simulink model "DCMotorSpeedControl_ClosedLoop"  (R2015b)
settings: Solver=VariableStepAuto  StartTime=0.0  StopTime=5  RelTol=1e-3
values from neighbouring files (symbols this model uses):
  Kv = (Vdc_nom - (I_nl*R_winding))/Om_nl    (= 0.00375385553259)    [MotorModel_Mabuchi_RS_540.m]    (also in Params.m = 0.0039)
  Vdc = 9.6    [MotorModel_Mabuchi_RS_540.m]    (also in Params.m)
libraries: LocalLib x2, simulink x1
settings Model: Creator=jje  LastModifiedBy=jje

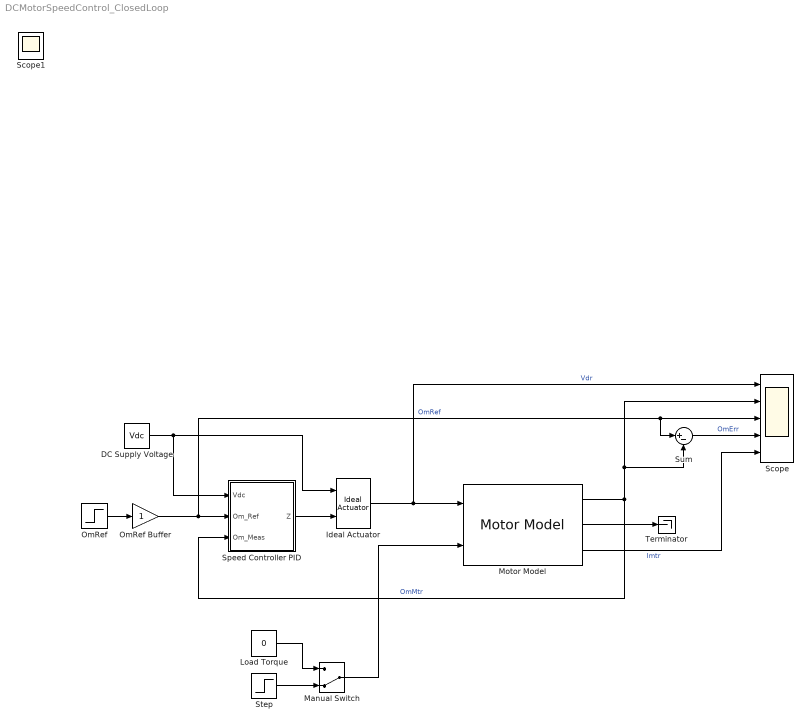
== system DCMotorSpeedControl_ClosedLoop ==
  DC Supply Voltage : Constant  Value=Vdc
  Ideal Actuator : LocalLib/Ideal Actuator
  Load Torque : Constant  Value=0
  Manual Switch : ManualSwitch  CurrentSetting=0
  Motor Model : LocalLib/Motor Model
  OmRef : Step  Time=0.01  After=10000*2*pi/60  SampleTime=0
  OmRef Buffer : Gain
  Scope : Scope  NumInputPorts=5
  Speed Controller PID : Subsystem
  Step : Step  Time=2  After=-0.1  SampleTime=0
  Sum : Sum  Inputs=|+-
  Terminator : Terminator
  Scope1 : Scope
  wires:
  DC Supply Voltage/1 -> Speed Controller PID/1(Vdc), Ideal Actuator/1
  Ideal Actuator/1 -> Motor Model/1, Scope/1  "Vdr"
  Motor Model/1 -> Speed Controller PID/3(Om_Meas), Sum/2, Scope/2  "OmMtr"
  Manual Switch/1 -> Motor Model/2
  OmRef/1 -> OmRef Buffer/1
  OmRef Buffer/1 -> Sum/1, Scope/3, Speed Controller PID/2(Om_Ref)  "OmRef"
  Sum/1 -> Scope/4  "OmErr"
  Motor Model/3 -> Scope/5  "Imtr"
  Motor Model/2 -> Terminator/1
  Speed Controller PID/1(Z) -> Ideal Actuator/2
  Load Torque/1 -> Manual Switch/1
  Step/1 -> Manual Switch/2

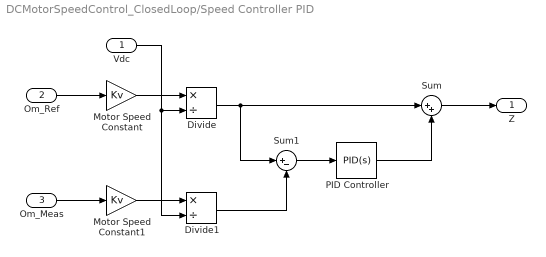
== system DCMotorSpeedControl_ClosedLoop/Speed Controller PID ==
  Vdc : Inport
  Om_Ref : Inport  Port=2
  Om_Meas : Inport  Port=3
  Divide : Product  Inputs=*/
  Divide1 : Product  Inputs=*/
  Motor Speed Constant : Gain  Gain=Kv
  Motor Speed Constant1 : Gain  Gain=Kv
  PID Controller : simulink/Continuous/PID Controller  Controller=PID  TimeDomain=Continuous-time  SampleTime=-1  IntegratorMethod=Forward Euler  FilterMethod=Forward Euler  Form=Ideal  UseFilter=on  ControllerParametersSource=internal  P=100  I=60  D=10  N=1  InitialConditionSource=internal  InitialConditionForIntegrator=0  InitialConditionForFilter=0  ExternalReset=none  LimitOutput=on  UpperSaturationLimit=1  LowerSaturationLimit=-1  LinearizeAsGain=on  AntiWindupMode=none  Kb=1  TrackingMode=off  Kt=1  PParamMin=[]  PParamMax=[]  IParamMin=[]  IParamMax=[]  DParamMin=[]  DParamMax=[]  NParamMin=[]  NParamMax=[]  KbParamMin=[]  KbParamMax=[]  KtParamMin=[]  KtParamMax=[]  POutMin=[]  POutMax=[]  IOutMin=[]  IOutMax=[]  DOutMin=[]  DOutMax=[]  NOutMin=[]  NOutMax=[]  KbOutMin=[]  KbOutMax=[]  KtOutMin=[]  KtOutMax=[]  IntegratorOutMin=[]  IntegratorOutMax=[]  FilterOutMin=[]  FilterOutMax=[]  SumOutMin=[]  SumOutMax=[]  SumI1OutMin=[]  SumI1OutMax=[]  SumI2OutMin=[]  SumI2OutMax=[]  SumI3OutMin=[]  SumI3OutMax=[]  SumDOutMin=[]  SumDOutMax=[]  SaturationOutMin=[]  SaturationOutMax=[]  IntegratorContinuousStateAttributes=''  IntegratorStateMustResolveToSignalObject=off  IntegratorRTWStateStorageClass=Auto  FilterContinuousStateAttributes=''  FilterStateMustResolveToSignalObject=off  FilterRTWStateStorageClass=Auto  DifferentiatorICPrevScaledInput=0  DifferentiatorOutMin=[]  DifferentiatorOutMax=[]
  Sum : Sum  Inputs=|++
  Sum1 : Sum  Inputs=|+-
  Z : Outport
  wires:
  Om_Ref/1 -> Motor Speed Constant/1
  Motor Speed Constant/1 -> Divide/1
  Vdc/1 -> Divide1/2, Divide/2
  Divide/1 -> Sum1/1, Sum/1
  Sum/1 -> Z/1
  Motor Speed Constant1/1 -> Divide1/1
  Om_Meas/1 -> Motor Speed Constant1/1
  Divide1/1 -> Sum1/2
  Sum1/1 -> PID Controller/1
  PID Controller/1 -> Sum/2
